simulink model "run_small_function"  (R2022b)
settings: Solver=VariableStepAuto  StartTime=0.0  StopTime=10.0  RelTol=1e-3
libraries: ece1718_small_function x5
settings Model: Creator=kevin  LastModifiedBy=kevin

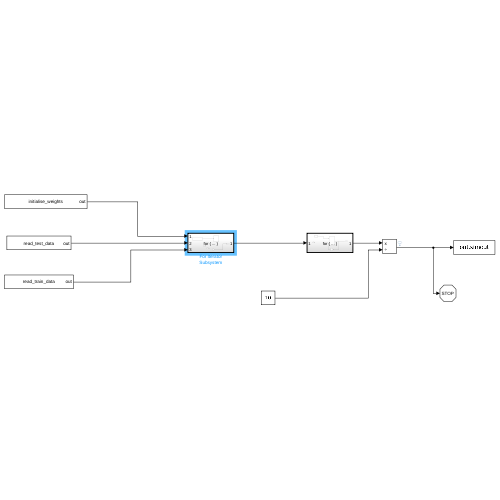
[thumbnail: Simulink's stored preview of the top-level diagram]
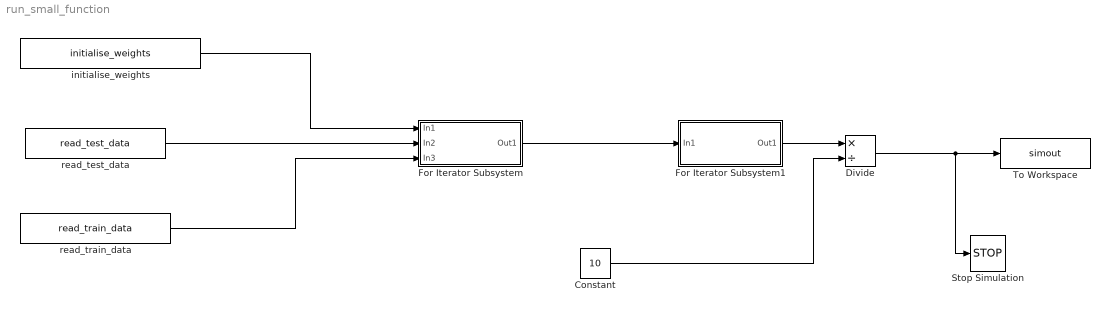
== system run_small_function ==
  Constant : Constant  Value=10
  Divide : Product  Inputs=*/  OutDataTypeStr=double
  For Iterator Subsystem : Subsystem  TreatAsAtomicUnit=on
  For Iterator Subsystem1 : Subsystem  TreatAsAtomicUnit=on
  Stop Simulation : Stop
  To Workspace : ToWorkspace  VariableName=simout  SaveFormat=Timeseries  SampleTime=-1
  initialise_weights : ece1718_small_function/initialise_weights  SampleTime=-1
      settings: SourceProductName=ece1718_small_function
  read_test_data : ece1718_small_function/read_test_data  SampleTime=-1
      settings: SourceProductName=ece1718_small_function
  read_train_data : ece1718_small_function/read_train_data  SampleTime=-1
      settings: SourceProductName=ece1718_small_function
  wires:
  For Iterator Subsystem/1(Out1) -> For Iterator Subsystem1/1(In1)
  read_test_data/1 -> For Iterator Subsystem/2(In2)
  read_train_data/1 -> For Iterator Subsystem/3(In3)
  For Iterator Subsystem1/1(Out1) -> Divide/1
  Constant/1 -> Divide/2
  Divide/1 -> Stop Simulation/1, To Workspace/1
  initialise_weights/1 -> For Iterator Subsystem/1(In1)

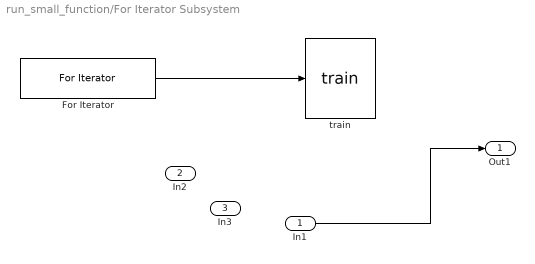
== system run_small_function/For Iterator Subsystem ==
  In1 : Inport
  In2 : Inport  Port=2
  In3 : Inport  Port=3
  For Iterator : ForIterator  IterationLimit=500  IndexMode=Zero-based
  train : ece1718_small_function/train  SampleTime=-1
      settings: SourceProductName=ece1718_small_function
  Out1 : Outport
  wires:
  For Iterator/1 -> train/1
  In1/1 -> Out1/1

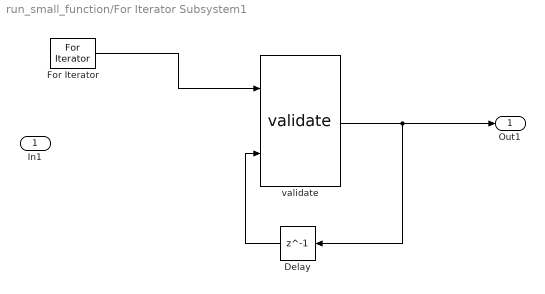
== system run_small_function/For Iterator Subsystem1 ==
  In1 : Inport
  Delay : Delay  DelayLength=1  InitialCondition=0
  For Iterator : ForIterator  IterationLimit=600  IndexMode=Zero-based
  validate : ece1718_small_function/validate  SampleTime=-1
      settings: SourceProductName=ece1718_small_function
  Out1 : Outport
  wires:
  validate/1 -> Delay/1, Out1/1
  For Iterator/1 -> validate/1
  Delay/1 -> validate/2
